simulink model "medium_microgrid_distribution_model"  (R2025b)
settings: Solver=ode23t  StartTime=0.0  StopTime=cfg.scenario.stop_time_s  MaxStep=1e-3  RelTol=1e-3
InitFcn:
  | if ~exist('cfg','var'), init_medium_microgrid; end
values from neighbouring files (symbols this model uses):
  cfg = init_medium_microgrid("grid_connected")    [create_medium_microgrid_model.m]    (also in init_medium_microgrid.m = struct(); run_medium_microgrid_scenarios.m = init_medium_microgrid(scenarioName))
undefined symbols (not defined in the file or in its folder): DiscIntNeverNeededParam
libraries: fl_lib x15, nesl_utility x9
settings Model: Creator=wang  LastModifiedBy=wang

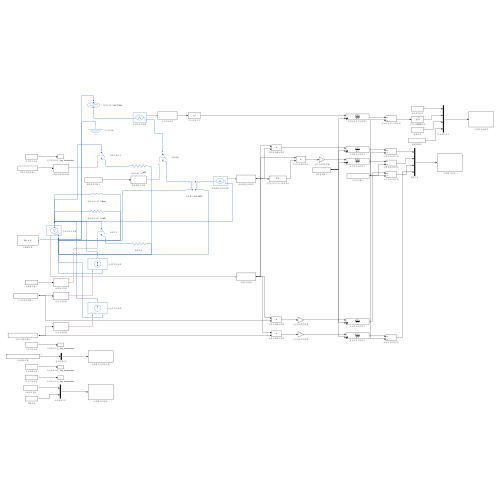
[thumbnail: Simulink's stored preview of the top-level diagram]
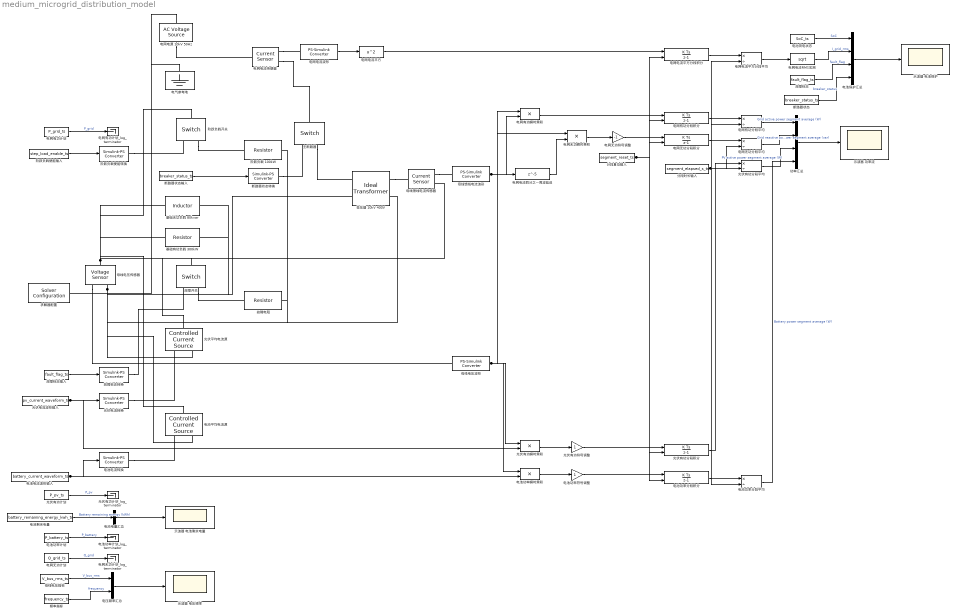
== system medium_microgrid_distribution_model ==
  主断路器 : fl_lib/Electrical/Electrical Elements/Switch  R_closed=0.01 Ohm  G_open=1e-8 1/Ohm  Threshold=0.5  i_specify=off  i_priority=None  i=0 A  i_nominal_specify=off  i_nominal_value=1  i_nominal_unit=A  v_specify=off  v_priority=None  v=0 V  v_nominal_specify=off  v_nominal_value=1  v_nominal_unit=V
  光伏平均电流源 : fl_lib/Electrical/Electrical Sources/Controlled Current Source
  光伏有功分段平均 : Product  Inputs=*/
  光伏有功分段积分 : DiscreteIntegrator  gainval=1  ExternalReset=rising  SampleTime=cfg.scenario.sample_time_s  ICPrevOutput=DiscIntNeverNeededParam  ICPrevScaledInput=DiscIntNeverNeededParam
  光伏有功瞬时乘积 : Product  Inputs=**
  光伏有功符号调整 : Gain
  光伏有功计划 : FromWorkspace  VariableName=P_pv_ts  SampleTime=cfg.scenario.sample_time_s
  光伏有功计划_log_terminator : Terminator
  光伏电流波形输入 : FromWorkspace  VariableName=pv_current_waveform_ts  SampleTime=cfg.scenario.sample_time_s
  光伏电流转换 : nesl_utility/Simulink-PS Converter  PhysicalDomain=network_engine_domain  SubClassName=ps_input  LeftPortType=input  RightPortType=output  PseudoPeriodic=off  Frequencies=[]  NoiseDistribution=none  NoiseParameters=[]  Unit=A  AffineConversion=off  FilteringAndDerivatives=provide  SimscapeFilterOrder=1  InputFilterTimeConstant=0.001  UdotUserProvided=0
  分段复位输入 : FromWorkspace  VariableName=segment_reset_ts  SampleTime=cfg.scenario.sample_time_s
  分段时长输入 : FromWorkspace  VariableName=segment_elapsed_s_ts  SampleTime=cfg.scenario.sample_time_s
  功率汇总 : Mux
  变压器 10kV 400V : fl_lib/Electrical/Electrical Elements/Ideal Transformer  n=cfg.transformer.turns_ratio  i1_specify=off  i1_priority=None  i1=0 A  i1_nominal_specify=off  i1_nominal_value=1  i1_nominal_unit=A  v1_specify=off  v1_priority=None  v1=0 V  v1_nominal_specify=off  v1_nominal_value=1  v1_nominal_unit=V  i2_specify=off  i2_priority=None  i2=0 A  i2_nominal_specify=off  i2_nominal_value=1  i2_nominal_unit=A  v2_specify=off  v2_priority=None  v2=0 V  v2_nominal_specify=off  v2_nominal_value=1  v2_nominal_unit=V
  基础无功负载 80kvar : fl_lib/Electrical/Electrical Elements/Inductor  l=cfg.load.base_inductance_h H  r=0 Ohm  g=1e-9 1/Ohm  i_specify=off  i_priority=None  i=0 A  i_nominal_specify=off  i_nominal_value=1  i_nominal_unit=A  v_specify=off  v_priority=None  v=0 V  v_nominal_specify=off  v_nominal_value=1  v_nominal_unit=V  i_L_specify=off  i_L_priority=High  i_L=0 A  i_L_nominal_specify=off  i_L_nominal_value=1  i_L_nominal_unit=A
  基础有功负载 300kW : fl_lib/Electrical/Electrical Elements/Resistor  R=cfg.load.base_resistance_ohm Ohm  i_specify=off  i_priority=None  i=0 A  i_nominal_specify=off  i_nominal_value=1  i_nominal_unit=A  v_specify=off  v_priority=None  v=0 V  v_nominal_specify=off  v_nominal_value=1  v_nominal_unit=V
  故障开关 : fl_lib/Electrical/Electrical Elements/Switch  R_closed=0.001 Ohm  G_open=1e-8 1/Ohm  Threshold=0.5  i_specify=off  i_priority=None  i=0 A  i_nominal_specify=off  i_nominal_value=1  i_nominal_unit=A  v_specify=off  v_priority=None  v=0 V  v_nominal_specify=off  v_nominal_value=1  v_nominal_unit=V
  故障标志 : FromWorkspace  VariableName=fault_flag_ts  SampleTime=cfg.scenario.sample_time_s
  故障标志转换 : nesl_utility/Simulink-PS Converter  PhysicalDomain=network_engine_domain  SubClassName=ps_input  LeftPortType=input  RightPortType=output  PseudoPeriodic=off  Frequencies=[]  NoiseDistribution=none  NoiseParameters=[]  Unit=1  AffineConversion=off  FilteringAndDerivatives=provide  SimscapeFilterOrder=1  InputFilterTimeConstant=0.001  UdotUserProvided=0
  故障标志输入 : FromWorkspace  VariableName=fault_flag_ts  SampleTime=cfg.scenario.sample_time_s
  故障电阻 : fl_lib/Electrical/Electrical Elements/Resistor  R=cfg.fault.resistance_ohm Ohm  i_specify=off  i_priority=None  i=0 A  i_nominal_specify=off  i_nominal_value=1  i_nominal_unit=A  v_specify=off  v_priority=None  v=0 V  v_nominal_specify=off  v_nominal_value=1  v_nominal_unit=V
  断路器状态 : FromWorkspace  VariableName=breaker_status_ts  SampleTime=cfg.scenario.sample_time_s
  断路器状态转换 : nesl_utility/Simulink-PS Converter  PhysicalDomain=network_engine_domain  SubClassName=ps_input  LeftPortType=input  RightPortType=output  PseudoPeriodic=off  Frequencies=[]  NoiseDistribution=none  NoiseParameters=[]  Unit=1  AffineConversion=off  FilteringAndDerivatives=provide  SimscapeFilterOrder=1  InputFilterTimeConstant=0.001  UdotUserProvided=0
  断路器状态输入 : FromWorkspace  VariableName=breaker_status_ts  SampleTime=cfg.scenario.sample_time_s
  母线电压传感器 : fl_lib/Electrical/Electrical Sensors/Voltage Sensor
  母线电压指标 : FromWorkspace  VariableName=V_bus_rms_ts  SampleTime=cfg.scenario.sample_time_s
  母线电压波形 : nesl_utility/PS-Simulink Converter  PhysicalDomain=network_engine_domain  SubClassName=ps_output  LeftPortType=input  RightPortType=output  PseudoPeriodic=off  Frequencies=[]  VectorFormat=inherit  Unit=V  AffineConversion=off
  母线馈线电流传感器 : fl_lib/Electrical/Electrical Sensors/Current Sensor
  母线馈线电流波形 : nesl_utility/PS-Simulink Converter  PhysicalDomain=network_engine_domain  SubClassName=ps_output  LeftPortType=input  RightPortType=output  PseudoPeriodic=off  Frequencies=[]  VectorFormat=inherit  Unit=A  AffineConversion=off
  求解器配置 : nesl_utility/Solver Configuration  PhysicalDomain=network_engine_domain  SubClassName=solver  LeftPortType=input  RightPortType=generic  Tones=[]  Harmonics=[]  SimulateNoise=off  Profile=off  UseLocalSampling=off  EnableSwitchedLinearOptims=on  FrequencyDomain=off  UseCCode=off  RelTol=0.001  AbsTol=0.001  MinStep=1e-09  ToWorkspace=off  RevertToSquareIcSolve=off  NumHomotopyIterations=100  PhasorMode=off  PhasorModeNumHarmonics=1  ConsistencySolver=NEWTON_XTOL_AFTER_FTOL  IndexReductionMethod=DerivativeReplacement  DoDC=off  ResidualTolerance=1e-09  ConsistencyTolSource=GLOBAL  ConsistencyAbsTol=0.001  ConsistencyRelTol=0.001  ConsistencyTolFactor=0.001  UseLocalSolver=off  LocalSolverChoice=NE_BACKWARD_EULER_ADVANCER  ResolveIndetEquations=on  FunctionEvalNumThread=1  LocalSolverSampleTime=0.001  DoFixedCost=off  MaxNonlinIter=3  MaxModeIter=2  ComputeImpulses=off  ImpulseIterations=2  LinearAlgebra=auto  LinearAlgebraNumThread=0  EquationFormulation=NE_TIME_EF  DelaysMemoryBudget=1024  AutomaticFiltering=on  FilteringTimeConstant=0.001  PartitionStorageMethod=AS_NEEDED  PartitionMemoryBudget=1024  PartitionMethod=ROBUST  MultibodyUseLocalSolver=off  MultibodyLocalSolverChoice=ODE1  MultibodyLocalSolverSampleTime=0.001
  电压频率汇总 : Mux  Inputs=2
  电气参考地 : fl_lib/Electrical/Electrical Elements/Electrical Reference
  电池保护汇总 : Mux
  电池剩余电量 : FromWorkspace  VariableName=battery_remaining_energy_kwh_ts  SampleTime=cfg.scenario.sample_time_s
  电池功率分段平均 : Product  Inputs=*/
  电池功率分段积分 : DiscreteIntegrator  gainval=1  ExternalReset=rising  SampleTime=cfg.scenario.sample_time_s  ICPrevOutput=DiscIntNeverNeededParam  ICPrevScaledInput=DiscIntNeverNeededParam
  电池功率瞬时乘积 : Product  Inputs=**
  电池功率符号调整 : Gain
  电池功率计划 : FromWorkspace  VariableName=P_battery_ts  SampleTime=cfg.scenario.sample_time_s
  电池功率计划_log_terminator : Terminator
  电池平均电流源 : fl_lib/Electrical/Electrical Sources/Controlled Current Source
  电池电流波形输入 : FromWorkspace  VariableName=battery_current_waveform_ts  SampleTime=cfg.scenario.sample_time_s
  电池电流转换 : nesl_utility/Simulink-PS Converter  PhysicalDomain=network_engine_domain  SubClassName=ps_input  LeftPortType=input  RightPortType=output  PseudoPeriodic=off  Frequencies=[]  NoiseDistribution=none  NoiseParameters=[]  Unit=A  AffineConversion=off  FilteringAndDerivatives=provide  SimscapeFilterOrder=1  InputFilterTimeConstant=0.001  UdotUserProvided=0
  电池电量汇总 : Mux  Inputs=1
  电池荷电状态 : FromWorkspace  VariableName=SoC_ts  SampleTime=cfg.scenario.sample_time_s
  电网无功分段平均 : Product  Inputs=*/
  电网无功分段积分 : DiscreteIntegrator  gainval=1  ExternalReset=rising  SampleTime=cfg.scenario.sample_time_s  ICPrevOutput=DiscIntNeverNeededParam  ICPrevScaledInput=DiscIntNeverNeededParam
  电网无功瞬时乘积 : Product  Inputs=**
  电网无功符号调整 : Gain  Gain=-1
  电网无功计划 : FromWorkspace  VariableName=Q_grid_ts  SampleTime=cfg.scenario.sample_time_s
  电网无功计划_log_terminator : Terminator
  电网有功分段平均 : Product  Inputs=*/
  电网有功分段积分 : DiscreteIntegrator  gainval=1  ExternalReset=rising  SampleTime=cfg.scenario.sample_time_s  ICPrevOutput=DiscIntNeverNeededParam  ICPrevScaledInput=DiscIntNeverNeededParam
  电网有功瞬时乘积 : Product  Inputs=**
  电网有功计划 : FromWorkspace  VariableName=P_grid_ts  SampleTime=cfg.scenario.sample_time_s
  电网有功计划_log_terminator : Terminator
  电网电流RMS实测 : Math  Operator=sqrt
  电网电流传感器 : fl_lib/Electrical/Electrical Sensors/Current Sensor
  电网电流四分之一周波延迟 : Delay  DelayLength=5  InitialCondition=0  SampleTime=cfg.scenario.sample_time_s
  电网电流平方 : Math  Operator=square
  电网电流平方分段平均 : Product  Inputs=*/
  电网电流平方分段积分 : DiscreteIntegrator  gainval=1  ExternalReset=rising  SampleTime=cfg.scenario.sample_time_s  ICPrevOutput=DiscIntNeverNeededParam  ICPrevScaledInput=DiscIntNeverNeededParam
  电网电流波形 : nesl_utility/PS-Simulink Converter  PhysicalDomain=network_engine_domain  SubClassName=ps_output  LeftPortType=input  RightPortType=output  PseudoPeriodic=off  Frequencies=[]  VectorFormat=inherit  Unit=A  AffineConversion=off
  电网电源 10kV 50Hz : fl_lib/Electrical/Electrical Sources/AC Voltage Source  amp=cfg.grid.primary_voltage_rms*sqrt(2) V  shift=0 deg  frequency=cfg.grid.frequency_hz Hz
  示波器 功率流 : Scope
  示波器 电压频率 : Scope
  示波器 电池保护 : Scope
  示波器 电池剩余电量 : Scope
  阶跃负载 100kW : fl_lib/Electrical/Electrical Elements/Resistor  R=cfg.load.step_resistance_ohm Ohm  i_specify=off  i_priority=None  i=0 A  i_nominal_specify=off  i_nominal_value=1  i_nominal_unit=A  v_specify=off  v_priority=None  v=0 V  v_nominal_specify=off  v_nominal_value=1  v_nominal_unit=V
  阶跃负载使能转换 : nesl_utility/Simulink-PS Converter  PhysicalDomain=network_engine_domain  SubClassName=ps_input  LeftPortType=input  RightPortType=output  PseudoPeriodic=off  Frequencies=[]  NoiseDistribution=none  NoiseParameters=[]  Unit=1  AffineConversion=off  FilteringAndDerivatives=provide  SimscapeFilterOrder=1  InputFilterTimeConstant=0.001  UdotUserProvided=0
  阶跃负载使能输入 : FromWorkspace  VariableName=step_load_enable_ts  SampleTime=cfg.scenario.sample_time_s
  阶跃负载开关 : fl_lib/Electrical/Electrical Elements/Switch  R_closed=0.01 Ohm  G_open=1e-8 1/Ohm  Threshold=0.5  i_specify=off  i_priority=None  i=0 A  i_nominal_specify=off  i_nominal_value=1  i_nominal_unit=A  v_specify=off  v_priority=None  v=0 V  v_nominal_specify=off  v_nominal_value=1  v_nominal_unit=V
  频率指标 : FromWorkspace  VariableName=frequency_ts  SampleTime=cfg.scenario.sample_time_s
  wires:
  光伏电流波形输入/1 -> 光伏有功瞬时乘积/2, 光伏电流转换/1
  电网有功分段积分/1 -> 电网有功分段平均/1
  电网有功计划/1 -> 电网有功计划_log_terminator/1  "P_grid"
  电网有功分段平均/1 -> 功率汇总/1  "Grid active power segment average (W)"
  阶跃负载使能输入/1 -> 阶跃负载使能转换/1
  光伏有功计划/1 -> 光伏有功计划_log_terminator/1  "P_pv"
  故障标志输入/1 -> 故障标志转换/1
  电池剩余电量/1 -> 电池电量汇总/1  "Battery remaining energy (kWh)"
  电池功率计划/1 -> 电池功率计划_log_terminator/1  "P_battery"
  频率指标/1 -> 电压频率汇总/2  "frequency"
  电池电流波形输入/1 -> 电池功率瞬时乘积/2, 电池电流转换/1
  电网无功计划/1 -> 电网无功计划_log_terminator/1  "Q_grid"
  母线电压指标/1 -> 电压频率汇总/1  "V_bus_rms"
  电网电流平方分段积分/1 -> 电网电流平方分段平均/1
  电池功率分段平均/1 -> 功率汇总/4  "Battery power segment average (W)"
  断路器状态/1 -> 电池保护汇总/4  "breaker_status"
  电池功率瞬时乘积/1 -> 电池功率符号调整/1
  电网电流RMS实测/1 -> 电池保护汇总/2  "I_grid_rms"
  电网电流平方/1 -> 电网电流平方分段积分/1
  电池电量汇总/1 -> 示波器 电池剩余电量/1
  分段时长输入/1 -> 电网有功分段平均/2, 电网电流平方分段平均/2, 光伏有功分段平均/2, 电网无功分段平均/2, 电池功率分段平均/2
  电压频率汇总/1 -> 示波器 电压频率/1
  断路器状态输入/1 -> 断路器状态转换/1
  分段复位输入/1 -> 电网电流平方分段积分/2, 电网无功分段积分/2, 电网有功分段积分/2, 光伏有功分段积分/2, 电池功率分段积分/2
  电网无功瞬时乘积/1 -> 电网无功符号调整/1
  母线电压波形/1 -> 电网无功瞬时乘积/1, 光伏有功瞬时乘积/1, 电网有功瞬时乘积/1, 电池功率瞬时乘积/1
  故障标志/1 -> 电池保护汇总/3  "fault_flag"
  电网电流波形/1 -> 电网电流平方/1
  母线馈线电流波形/1 -> 电网有功瞬时乘积/2, 电网电流四分之一周波延迟/1
  功率汇总/1 -> 示波器 功率流/1
  电网有功瞬时乘积/1 -> 电网有功分段积分/1
  电网电流四分之一周波延迟/1 -> 电网无功瞬时乘积/2
  光伏有功瞬时乘积/1 -> 光伏有功符号调整/1
  光伏有功符号调整/1 -> 光伏有功分段积分/1
  电池功率符号调整/1 -> 电池功率分段积分/1
  电网无功符号调整/1 -> 电网无功分段积分/1
  电网无功分段积分/1 -> 电网无功分段平均/1
  电网电流平方分段平均/1 -> 电网电流RMS实测/1
  光伏有功分段积分/1 -> 光伏有功分段平均/1
  电池功率分段积分/1 -> 电池功率分段平均/1
  电网无功分段平均/1 -> 功率汇总/2  "Grid reactive power segment average (var)"
  光伏有功分段平均/1 -> 功率汇总/3  "PV active power segment average (W)"
  电池荷电状态/1 -> 电池保护汇总/1  "SoC"
  电池保护汇总/1 -> 示波器 电池保护/1
  connections:
  电网电源 10kV 50Hz/RConn1 -- 电网电流传感器/LConn1
  阶跃负载使能转换/RConn1 -- 阶跃负载开关/RConn1
  主断路器/RConn2 -- 变压器 10kV 400V/LConn1
  母线电压传感器/RConn2 -- 求解器配置/RConn1 -- 电网电源 10kV 50Hz/LConn1 -- 电气参考地/LConn1 -- 光伏平均电流源/RConn2 -- 基础有功负载 300kW/RConn1 -- 基础无功负载 80kvar/RConn1 -- 变压器 10kV 400V/LConn2 -- 故障电阻/RConn1 -- 电池平均电流源/RConn2 -- 变压器 10kV 400V/RConn2 -- 阶跃负载 100kW/RConn1
  母线电压传感器/RConn1 -- 母线电压波形/LConn1
  母线电压传感器/LConn1 -- 故障开关/LConn1 -- 基础无功负载 80kvar/LConn1 -- 光伏平均电流源/LConn1 -- 阶跃负载开关/LConn1 -- 母线馈线电流传感器/RConn2 -- 电池平均电流源/LConn1 -- 基础有功负载 300kW/LConn1
  故障标志转换/RConn1 -- 故障开关/RConn1
  光伏电流转换/RConn1 -- 光伏平均电流源/RConn1
  电池电流转换/RConn1 -- 电池平均电流源/RConn1
  阶跃负载开关/RConn2 -- 阶跃负载 100kW/LConn1
  故障开关/RConn2 -- 故障电阻/LConn1
  电网电流传感器/RConn1 -- 电网电流波形/LConn1
  电网电流传感器/RConn2 -- 主断路器/LConn1
  断路器状态转换/RConn1 -- 主断路器/RConn1
  变压器 10kV 400V/RConn1 -- 母线馈线电流传感器/LConn1
  母线馈线电流传感器/RConn1 -- 母线馈线电流波形/LConn1
